simulink model "new_nncontroller_3_50"  (R2021a)
settings: Solver=VariableStepAuto  StartTime=0.0  StopTime=10.0  RelTol=1e-3
libraries: neural x155
(part 8 of 8)

== system new_nncontroller_3_50/Feed-Forward Neural Network/Layer 4/Delays 1 ==
  "p{4}" : Inport  PortDimensions=50
      mask Display: e = 0.06;c1 = [120 230 180]/255;c2 = ([120 230 180]+0)/(256+128);c3 = ([120 230 180]+128)/(256+128);patch([0 1 1 0],[0 0 1 1],c1);patch([0 1 1 1-e 1-e 0+e],[0 0 1 1-e 0+e 0+e],c2);patch([0 0 1 1-e 0+e 0+e],[0 1 1 1-e 1-e 0+e],c3);plot([0 1 1 0 0],[0 0 1 1 0]);
  mux : Mux  Inputs=1
      mask Display: e = 0.06;c1 = [120 150 230]/255;c2 = ([120 150 230]+0)/383;c3 = ([120 150 230]+128)/383;patch([0 1 1 0],[0 0 1 1],c1);patch([0 1 1 1-e 1-e 0+e],[0 0 1 1-e 0+e 0+e],c2);patch([0 0 1 1-e 0+e 0+e],[0 1 1 1-e 1-e 0+e],c3);plot([0 1 1 0 0],[0 0 1 1 0]);disp('Mux')
  "pd{4,3}" : Outport
      mask Display: e = 0.06;c1 = [120 230 180]/255;c2 = ([120 230 180]+0)/(256+128);c3 = ([120 230 180]+128)/(256+128);patch([0 1 1 0],[0 0 1 1],c1);patch([0 1 1 1-e 1-e 0+e],[0 0 1 1-e 0+e 0+e],c2);patch([0 0 1 1-e 0+e 0+e],[0 1 1 1-e 1-e 0+e],c3);plot([0 1 1 0 0],[0 0 1 1 0]);
  wires:
  "p{4}"/1 -> mux/1
  mux/1 -> "pd{4,3}"/1

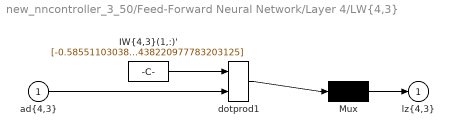
== system new_nncontroller_3_50/Feed-Forward Neural Network/Layer 4/LW{4,3} ==
  "ad{4,3}" : Inport  PortDimensions=50
      mask Display: e = 0.06;c1 = [120 230 180]/255;c2 = ([120 230 180]+0)/(256+128);c3 = ([120 230 180]+128)/(256+128);patch([0 1 1 0],[0 0 1 1],c1);patch([0 1 1 1-e 1-e 0+e],[0 0 1 1-e 0+e 0+e],c2);patch([0 0 1 1-e 0+e 0+e],[0 1 1 1-e 1-e 0+e],c3);plot([0 1 1 0 0],[0 0 1 1 0]);
  "IW{4,3}(1,:)'" : Constant  Value=[-0.58551103038991569871285491899470798671245574951171875;-0.289105065397524452208699585753493010997772216796875;0.216777904259323694891037348497775383293628692626953125;0.3397660222592506773509057893534190952777862548828125;0.4508963301912753962596980272792279720306396484375;-0.07590620785706279904925253276815055869519710540771484375;0.193753389454290603222119671045220457017421722412109375;-0.9347152745077933477801934714079834520816802978515625;-0.2117256694345168721582695070537738502025604248046875;0.31554249414756885272481667925603687763214111328125;-0.400781938442792640131528969504870474338531494140625;0.9820194374011343985131361478124745190143585205078125;-0.7015966116216045822540081644547171890735626220703125;0.97416360982369598620067563388147391378879547119140625;-0.00856368652055551626833818090744898654520511627197265625;0.872760775509000108485224700416438281536102294921875;-0.332117999106419092836262052514939568936824798583984375;0.0494382022691290945459741124068386852741241455078125;0.018723337834972118842724597698179422877728939056396484375;0.60343009635602629092687720913090743124485015869140625;-0.8762731163601664707840654955361969769001007080078125;0.1207058317122336188464970518907648511230945587158203125;0.640630117487245964724706936976872384548187255859375;0.347470955628215616428633438772521913051605224609375;-0.71973069539375800207636757477303035557270050048828125;0.3008516484234269316999643706367351114749908447265625;0.329625798000043823687832400537445209920406341552734375;0.96656540211900232595354509612661786377429962158203125;0.79590336830352714780900669211405329406261444091796875;-0.674134029669995360478651491575874388217926025390625;-0.014789801065709706762163477833382785320281982421875;0.60401660798405887309314721278497017920017242431640625;-0.390510945954118116052455889075645245611667633056640625;-0.35643095258122536872491536996676586568355560302734375;-0.146763640045544152545886618099757470190525054931640625;0.34021410623316505894564443224226124584674835205078125;-0.47747852096776444152936846876400522887706756591796875;-0.0846525835835105766591368592344224452972412109375;-0.59369403811485976785178309000912122428417205810546875;-0.152411797296135465007438369866576977074146270751953125;-0.281285239152872457157883445688639767467975616455078125;-0.0975028564320883361915548448450863361358642578125;-0.356807400209386560430147028455394320189952850341796875;0.549797831237108791668788398965261876583099365234375;-0.17248927525704260688144131563603878021240234375;-0.0457572011023563707254879773245193064212799072265625;0.07153366761153230612979569968956639058887958526611328125;-0.54516397156672102841667992834118194878101348876953125;0.8371955028115014574296992577728815376758575439453125;0.5422048464022719560517771242302842438220977783203125]
      mask Display: e = 0.06;c1 = [120 150 230]/255;c2 = ([120 150 230]+0)/383;c3 = ([120 150 230]+128)/383;patch([0 1 1 0],[0 0 1 1],c1);patch([0 1 1 1-e 1-e 0+e],[0 0 1 1-e 0+e 0+e],c2);patch([0 0 1 1-e 0+e 0+e],[0 1 1 1-e 1-e 0+e],c3);plot([0 1 1 0 0],[0 0 1 1 0]);disp('weights');
  Mux : Mux  Inputs=1
      mask Display: e = 0.06;c1 = [120 150 230]/255;c2 = ([120 150 230]+0)/383;c3 = ([120 150 230]+128)/383;patch([0 1 1 0],[0 0 1 1],c1);patch([0 1 1 1-e 1-e 0+e],[0 0 1 1-e 0+e 0+e],c2);patch([0 0 1 1-e 0+e 0+e],[0 1 1 1-e 1-e 0+e],c3);plot([0 1 1 0 0],[0 0 1 1 0]);disp('Mux');
  dotprod1 : neural/Weight Functions/dotprod
  "lz{4,3}" : Outport
      mask Display: e = 0.06;c1 = [120 230 180]/255;c2 = ([120 230 180]+0)/(256+128);c3 = ([120 230 180]+128)/(256+128);patch([0 1 1 0],[0 0 1 1],c1);patch([0 1 1 1-e 1-e 0+e],[0 0 1 1-e 0+e 0+e],c2);patch([0 0 1 1-e 0+e 0+e],[0 1 1 1-e 1-e 0+e],c3);plot([0 1 1 0 0],[0 0 1 1 0]);
  wires:
  "IW{4,3}(1,:)'"/1 -> dotprod1/1
  "ad{4,3}"/1 -> dotprod1/2
  dotprod1/1 -> Mux/1
  Mux/1 -> "lz{4,3}"/1
